simulink model "admittance_control"  (R2020b)
settings: Solver=VariableStepAuto  StartTime=0.0  StopTime=9.3  RelTol=1e-3
values from neighbouring files (symbols this model uses):
  assis = 0.5    [admittance.m]
  emg_ratio = 0    [admittance.m]
  ext = 0.2    [admittance.m]
  h_stiff = 5    [admittance.m]
  help_op = -1    [admittance.m]
  l_stiff = 2    [admittance.m]
  walk = 1    [admittance.m]
libraries: pid_lib x3
settings Model: Creator=montano  LastModifiedBy=Carlos

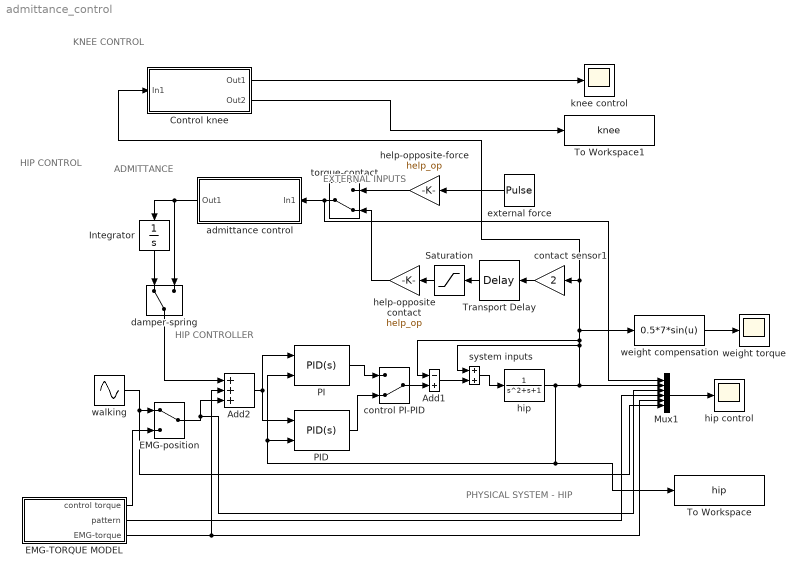
== system admittance_control ==
  note: HIP CONTROL
  note: EXTERNAL INPUTS
  note: KNEE CONTROL
  note: ADMITTANCE
  note: HIP CONTROLLER
  note: PHYSICAL SYSTEM - HIP
  Add1 : Sum  Inputs=-+
  Add2 : Sum  Inputs=+++
  Control knee : Subsystem
  EMG-TORQUE MODEL : Subsystem
  EMG-position : ManualSwitch
  Integrator : Integrator
  Mux1 : Mux  Inputs=6
  PI : pid_lib/PID Controller (2DOF)  Controller=PID  Form=Parallel  TimeDomain=Continuous-time  UseExternalTs=off  SampleTime=-1  IntegratorMethod=Forward Euler  FilterMethod=Forward Euler  ControllerParametersSource=internal  P=200  I=1  D=0  UseFilter=on  N=100  b=1  c=1  TunerSelectOption=Transfer Function Based (PID Tuner App)  InitialConditionSource=internal  InitialConditionForIntegrator=0  InitialConditionForFilter=0  DifferentiatorICPrevScaledInput=0  ExternalReset=none  TrackingMode=off  Kt=1  LimitOutput=off  SatLimitsSource=internal  UpperSaturationLimit=inf  LowerSaturationLimit=-inf  LinearizeAsGain=on  AntiWindupMode=none  Kb=1  POutMin=[]  POutMax=[]  IOutMin=[]  IOutMax=[]  DOutMin=[]  DOutMax=[]  NOutMin=[]  NOutMax=[]  bOutMin=[]  bOutMax=[]  cOutMin=[]  cOutMax=[]  SumOutMin=[]  SumOutMax=[]  SaturationOutMin=[]  SaturationOutMax=[]  PParamMin=[]  PParamMax=[]  IParamMin=[]  IParamMax=[]  DParamMin=[]  DParamMax=[]  NParamMin=[]  NParamMax=[]  bParamMin=[]  bParamMax=[]  cParamMin=[]  cParamMax=[]  KbParamMin=[]  KbParamMax=[]  KtParamMin=[]  KtParamMax=[]  KbOutMin=[]  KbOutMax=[]  KtOutMin=[]  KtOutMax=[]  IntegratorOutMin=[]  IntegratorOutMax=[]  FilterOutMin=[]  FilterOutMax=[]  SumI1OutMin=[]  SumI1OutMax=[]  SumI2OutMin=[]  SumI2OutMax=[]  SumI3OutMin=[]  SumI3OutMax=[]  SumI4OutMin=[]  SumI4OutMax=[]  SumDOutMin=[]  SumDOutMax=[]  Sum1OutMin=[]  Sum1OutMax=[]  Sum2OutMin=[]  Sum2OutMax=[]  Sum3OutMin=[]  Sum3OutMax=[]  DifferentiatorOutMin=[]  DifferentiatorOutMax=[]  FilterDiffOutCoefMin=[]  FilterDiffOutCoefMax=[]  ReciprocalOutMin=[]  ReciprocalOutMax=[]  SumDenOutMin=[]  SumDenOutMax=[]  SumNumOutMin=[]  SumNumOutMax=[]  DivideOutMin=[]  DivideOutMax=[]  UdiffTsProdOutMin=[]  UdiffTsProdOutMax=[]  NTsProdOutMin=[]  NTsProdOutMax=[]  UintegralTsProdOutMin=[]  UintegralTsProdOutMax=[]  UngainTsProdOutMin=[]  UngainTsProdOutMax=[]  IntegratorContinuousStateAttributes=''  IntegratorStateMustResolveToSignalObject=off  IntegratorRTWStateStorageClass=Auto  FilterContinuousStateAttributes=''  FilterStateMustResolveToSignalObject=off  FilterRTWStateStorageClass=Auto  ParallelPVariant=InternalParameters  IdealPVariant=Disabled  IVariant=InternalParameters  DVariant=InternalParameters  bVariant=InternalParameters  cVariant=InternalParameters  IntegratorVariant=Continuous  SatVariant=Disabled  AWVariant=Passthrough  PCopyVariant=Disabled  TRVariant=Disabled  FdbkBlocksVariant=Forward  IdealPFdbkVariant=Disabled  SatFdbkVariant=Disabled  DerivativeFilterVariant=ContFilter  NVariant=InternalParameters  NCopyVariant=Disabled  FilterICVariant=InternalICsFilter  IntegratorICVariant=InternalICs  ExternalResetVariant=Disabled  TRSumVariant=Passthrough  SumFdbkVariant=Disabled  SumVariant=Sum_PID  TsampFilterVariant=InternalTs  TsampNgainVariant=Passthrough  TsampIntegralVariant=Passthrough  ExternalSaturationOutDataTypeStr=Inherit: Same as second input
      settings: SourceProductBaseCode=SL
  PID : pid_lib/PID Controller (2DOF)  Controller=PID  Form=Parallel  TimeDomain=Continuous-time  UseExternalTs=off  SampleTime=-1  IntegratorMethod=Forward Euler  FilterMethod=Forward Euler  ControllerParametersSource=internal  P=200  I=1  D=10  UseFilter=on  N=100  b=1  c=1  TunerSelectOption=Transfer Function Based (PID Tuner App)  InitialConditionSource=internal  InitialConditionForIntegrator=0  InitialConditionForFilter=0  DifferentiatorICPrevScaledInput=0  ExternalReset=none  TrackingMode=off  Kt=1  LimitOutput=off  SatLimitsSource=internal  UpperSaturationLimit=inf  LowerSaturationLimit=-inf  LinearizeAsGain=on  AntiWindupMode=none  Kb=1  POutMin=[]  POutMax=[]  IOutMin=[]  IOutMax=[]  DOutMin=[]  DOutMax=[]  NOutMin=[]  NOutMax=[]  bOutMin=[]  bOutMax=[]  cOutMin=[]  cOutMax=[]  SumOutMin=[]  SumOutMax=[]  SaturationOutMin=[]  SaturationOutMax=[]  PParamMin=[]  PParamMax=[]  IParamMin=[]  IParamMax=[]  DParamMin=[]  DParamMax=[]  NParamMin=[]  NParamMax=[]  bParamMin=[]  bParamMax=[]  cParamMin=[]  cParamMax=[]  KbParamMin=[]  KbParamMax=[]  KtParamMin=[]  KtParamMax=[]  KbOutMin=[]  KbOutMax=[]  KtOutMin=[]  KtOutMax=[]  IntegratorOutMin=[]  IntegratorOutMax=[]  FilterOutMin=[]  FilterOutMax=[]  SumI1OutMin=[]  SumI1OutMax=[]  SumI2OutMin=[]  SumI2OutMax=[]  SumI3OutMin=[]  SumI3OutMax=[]  SumI4OutMin=[]  SumI4OutMax=[]  SumDOutMin=[]  SumDOutMax=[]  Sum1OutMin=[]  Sum1OutMax=[]  Sum2OutMin=[]  Sum2OutMax=[]  Sum3OutMin=[]  Sum3OutMax=[]  DifferentiatorOutMin=[]  DifferentiatorOutMax=[]  FilterDiffOutCoefMin=[]  FilterDiffOutCoefMax=[]  ReciprocalOutMin=[]  ReciprocalOutMax=[]  SumDenOutMin=[]  SumDenOutMax=[]  SumNumOutMin=[]  SumNumOutMax=[]  DivideOutMin=[]  DivideOutMax=[]  UdiffTsProdOutMin=[]  UdiffTsProdOutMax=[]  NTsProdOutMin=[]  NTsProdOutMax=[]  UintegralTsProdOutMin=[]  UintegralTsProdOutMax=[]  UngainTsProdOutMin=[]  UngainTsProdOutMax=[]  IntegratorContinuousStateAttributes=''  IntegratorStateMustResolveToSignalObject=off  IntegratorRTWStateStorageClass=Auto  FilterContinuousStateAttributes=''  FilterStateMustResolveToSignalObject=off  FilterRTWStateStorageClass=Auto  ParallelPVariant=InternalParameters  IdealPVariant=Disabled  IVariant=InternalParameters  DVariant=InternalParameters  bVariant=InternalParameters  cVariant=InternalParameters  IntegratorVariant=Continuous  SatVariant=Disabled  AWVariant=Passthrough  PCopyVariant=Disabled  TRVariant=Disabled  FdbkBlocksVariant=Forward  IdealPFdbkVariant=Disabled  SatFdbkVariant=Disabled  DerivativeFilterVariant=ContFilter  NVariant=InternalParameters  NCopyVariant=Disabled  FilterICVariant=InternalICsFilter  IntegratorICVariant=InternalICs  ExternalResetVariant=Disabled  TRSumVariant=Passthrough  SumFdbkVariant=Disabled  SumVariant=Sum_PID  TsampFilterVariant=InternalTs  TsampNgainVariant=Passthrough  TsampIntegralVariant=Passthrough  ExternalSaturationOutDataTypeStr=Inherit: Same as second input
      settings: SourceProductBaseCode=SL
  Saturation : Saturate  UpperLimit=1  LowerLimit=0
  To Workspace : ToWorkspace  VariableName=hip  SampleTime=-1
  To Workspace1 : ToWorkspace  VariableName=knee  SampleTime=-1
  Transport Delay : TransportDelay  DelayTime=5.25
  admittance control : Subsystem
  contact sensor1 : Gain  Gain=2
  control PI-PID : ManualSwitch  CurrentSetting=0
  damper-spring : ManualSwitch
  external force : DiscretePulseGenerator  PulseType=Time based  Amplitude=ext  Period=10  PulseWidth=25  PhaseDelay=2
  help-opposite contact : Gain  Gain=help_op
  help-opposite-force : Gain  Gain=help_op
  hip : TransferFcn  Denominator=[1 1 1]
  "hip control " : Scope
  knee control : Scope
  system inputs : Sum
  torque-contact : ManualSwitch  CurrentSetting=0
  walking : Sin  Amplitude=walk  Frequency=2.4  SampleTime=0
  weight compensation : MATLABFcn  MATLABFcn=0.5*7*sin(u)
  weight torque : Scope
  wires:
  Mux1/1 -> "hip control "/1
  hip/1 -> PI/2, PID/2, To Workspace/1, Control knee/1(In1), contact sensor1/1, weight compensation/1, Add1/1, system inputs/1, Mux1/2
  Add2/1 -> PI/1, PID/1
  Transport Delay/1 -> Saturation/1
  contact sensor1/1 -> Transport Delay/1
  PID/1 -> control PI-PID/2
  PI/1 -> control PI-PID/1
  Control knee/1(Out1) -> knee control/1
  admittance control/1(Out1) -> Integrator/1, damper-spring/2
  torque-contact/1 -> admittance control/1(In1), Mux1/1
  Control knee/2(Out2) -> To Workspace1/1
  Integrator/1 -> damper-spring/1
  Saturation/1 -> help-opposite contact/1
  help-opposite contact/1 -> torque-contact/2
  external force/1 -> help-opposite-force/1
  help-opposite-force/1 -> torque-contact/1
  EMG-TORQUE MODEL/2(pattern) -> Mux1/4
  walking/1 -> Mux1/6, EMG-position/1
  EMG-TORQUE MODEL/1(control torque) -> EMG-position/2
  EMG-TORQUE MODEL/3(EMG-torque) -> Add2/2, Mux1/5
  EMG-position/1 -> Add2/3, Mux1/3
  weight compensation/1 -> weight torque/1
  damper-spring/1 -> Add2/1
  control PI-PID/1 -> Add1/2
  Add1/1 -> system inputs/2
  system inputs/1 -> hip/1

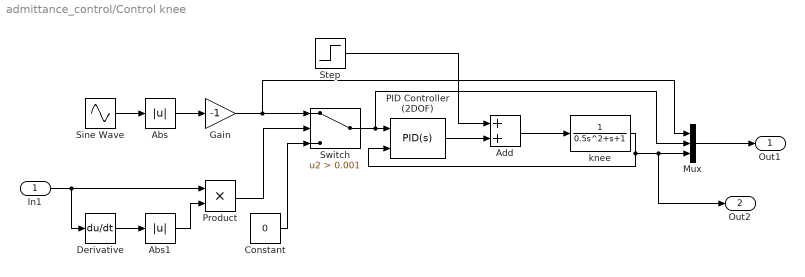
== system admittance_control/Control knee ==
  In1 : Inport
  Abs : Abs
  Abs1 : Abs
  Add : Sum
  Constant : Constant  Value=0
  Derivative : Derivative
  Gain : Gain  Gain=-1
  Mux : Mux  Inputs=3
  PID Controller (2DOF) : pid_lib/PID Controller (2DOF)  Controller=PID  Form=Parallel  TimeDomain=Continuous-time  UseExternalTs=off  SampleTime=-1  IntegratorMethod=Forward Euler  FilterMethod=Forward Euler  ControllerParametersSource=internal  P=18  I=10  D=10  UseFilter=on  N=100  b=1  c=1  TunerSelectOption=Transfer Function Based (PID Tuner App)  InitialConditionSource=internal  InitialConditionForIntegrator=0  InitialConditionForFilter=0  DifferentiatorICPrevScaledInput=0  ExternalReset=none  TrackingMode=off  Kt=1  LimitOutput=off  SatLimitsSource=internal  UpperSaturationLimit=inf  LowerSaturationLimit=-inf  LinearizeAsGain=on  AntiWindupMode=none  Kb=1  POutMin=[]  POutMax=[]  IOutMin=[]  IOutMax=[]  DOutMin=[]  DOutMax=[]  NOutMin=[]  NOutMax=[]  bOutMin=[]  bOutMax=[]  cOutMin=[]  cOutMax=[]  SumOutMin=[]  SumOutMax=[]  SaturationOutMin=[]  SaturationOutMax=[]  PParamMin=[]  PParamMax=[]  IParamMin=[]  IParamMax=[]  DParamMin=[]  DParamMax=[]  NParamMin=[]  NParamMax=[]  bParamMin=[]  bParamMax=[]  cParamMin=[]  cParamMax=[]  KbParamMin=[]  KbParamMax=[]  KtParamMin=[]  KtParamMax=[]  KbOutMin=[]  KbOutMax=[]  KtOutMin=[]  KtOutMax=[]  IntegratorOutMin=[]  IntegratorOutMax=[]  FilterOutMin=[]  FilterOutMax=[]  SumI1OutMin=[]  SumI1OutMax=[]  SumI2OutMin=[]  SumI2OutMax=[]  SumI3OutMin=[]  SumI3OutMax=[]  SumI4OutMin=[]  SumI4OutMax=[]  SumDOutMin=[]  SumDOutMax=[]  Sum1OutMin=[]  Sum1OutMax=[]  Sum2OutMin=[]  Sum2OutMax=[]  Sum3OutMin=[]  Sum3OutMax=[]  DifferentiatorOutMin=[]  DifferentiatorOutMax=[]  FilterDiffOutCoefMin=[]  FilterDiffOutCoefMax=[]  ReciprocalOutMin=[]  ReciprocalOutMax=[]  SumDenOutMin=[]  SumDenOutMax=[]  SumNumOutMin=[]  SumNumOutMax=[]  DivideOutMin=[]  DivideOutMax=[]  UdiffTsProdOutMin=[]  UdiffTsProdOutMax=[]  NTsProdOutMin=[]  NTsProdOutMax=[]  UintegralTsProdOutMin=[]  UintegralTsProdOutMax=[]  UngainTsProdOutMin=[]  UngainTsProdOutMax=[]  IntegratorContinuousStateAttributes=''  IntegratorStateMustResolveToSignalObject=off  IntegratorRTWStateStorageClass=Auto  FilterContinuousStateAttributes=''  FilterStateMustResolveToSignalObject=off  FilterRTWStateStorageClass=Auto  ParallelPVariant=InternalParameters  IdealPVariant=Disabled  IVariant=InternalParameters  DVariant=InternalParameters  bVariant=InternalParameters  cVariant=InternalParameters  IntegratorVariant=Continuous  SatVariant=Disabled  AWVariant=Passthrough  PCopyVariant=Disabled  TRVariant=Disabled  FdbkBlocksVariant=Forward  IdealPFdbkVariant=Disabled  SatFdbkVariant=Disabled  DerivativeFilterVariant=ContFilter  NVariant=InternalParameters  NCopyVariant=Disabled  FilterICVariant=InternalICsFilter  IntegratorICVariant=InternalICs  ExternalResetVariant=Disabled  TRSumVariant=Passthrough  SumFdbkVariant=Disabled  SumVariant=Sum_PID  TsampFilterVariant=InternalTs  TsampNgainVariant=Passthrough  TsampIntegralVariant=Passthrough  ExternalSaturationOutDataTypeStr=Inherit: Same as second input
      settings: SourceProductBaseCode=SL
  Product : Product
  Sine Wave : Sin  Amplitude=0.5  Frequency=2.4  SampleTime=0
  Step : Step  Time=5  After=0  SampleTime=0
  Switch : Switch  Criteria=u2 > Threshold  Threshold=0.001
  "knee " : TransferFcn  Denominator=[0.5 1 1]
  Out1 : Outport
  Out2 : Outport  Port=2
  wires:
  Mux/1 -> Out1/1
  "knee "/1 -> Out2/1, Mux/3, PID Controller (2DOF)/2
  Constant/1 -> Switch/3
  PID Controller (2DOF)/1 -> Add/2
  Step/1 -> Add/1
  Add/1 -> "knee "/1
  Switch/1 -> Mux/2, PID Controller (2DOF)/1
  In1/1 -> Product/1, Derivative/1
  Sine Wave/1 -> Abs/1
  Derivative/1 -> Abs1/1
  Abs1/1 -> Product/2
  Product/1 -> Switch/2
  Abs/1 -> Gain/1
  Gain/1 -> Mux/1, Switch/1

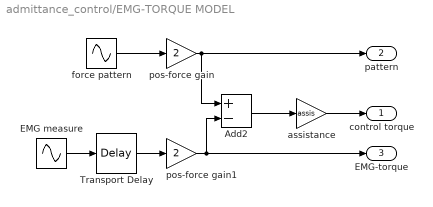
== system admittance_control/EMG-TORQUE MODEL ==
  Add2 : Sum  Inputs=+-
  EMG measure : Sin  Amplitude=0.35*emg_ratio  Frequency=2.4  SampleTime=0
  Transport Delay : TransportDelay  DelayTime=0
  assistance : Gain  Gain=assis
  force pattern : Sin  Amplitude=0.35  Frequency=2.4  SampleTime=0
  pos-force gain : Gain  Gain=2
  pos-force gain1 : Gain  Gain=2
  control torque : Outport
  pattern : Outport  Port=2
  EMG-torque : Outport  Port=3
  wires:
  force pattern/1 -> pos-force gain/1
  pos-force gain/1 -> pattern/1, Add2/1
  pos-force gain1/1 -> EMG-torque/1, Add2/2
  Add2/1 -> assistance/1
  assistance/1 -> control torque/1
  EMG measure/1 -> Transport Delay/1
  Transport Delay/1 -> pos-force gain1/1

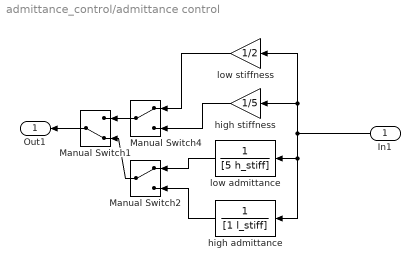
== system admittance_control/admittance control ==
  In1 : Inport
  Manual Switch1 : ManualSwitch  CurrentSetting=0
  Manual Switch2 : ManualSwitch
  Manual Switch4 : ManualSwitch
  high admittance : TransferFcn  Numerator=1  Denominator=[1 l_stiff]
  high stiffness : Gain  Gain=1/5
  low admittance : TransferFcn  Denominator=[5 h_stiff]
  low stiffness : Gain  Gain=1/2
  Out1 : Outport
  wires:
  Manual Switch4/1 -> Manual Switch1/1
  In1/1 -> low stiffness/1, high stiffness/1, low admittance/1, high admittance/1
  Manual Switch2/1 -> Manual Switch1/2
  high stiffness/1 -> Manual Switch4/2
  low stiffness/1 -> Manual Switch4/1
  high admittance/1 -> Manual Switch2/2
  low admittance/1 -> Manual Switch2/1
  Manual Switch1/1 -> Out1/1
